simulink model "my_macro_2_2025"  (R2026a)
settings: Solver=VariableStepAuto
values from neighbouring files (symbols this model uses):
  A = [A_init, zeros(5,1) ... (first row only)    [IP_MACRO.m]    (also in testes_30_03.m)
  A_c = [A - B*K - L*C,  -B*K_i ... (first row only)    [Home1.m]
  B = [B_init ... (first row only)    [IP_MACRO.m]    (also in testes_30_03.m)
  B_c = [L ... (first row only)    [Home1.m]
  C = [C_init, zeros(2,1)]    [IP_MACRO.m]    (also in testes_30_03.m)
  C_c = -K_aug    [Home1.m]
  D = zeros(2,1)    [IP_MACRO.m]    (also in testes_30_03.m)
  D_c = [0, 0]    [Home1.m]
  x0 = [0.1 0 0.05 0 0]'    [Home1.m]
settings Model: Creator=sofia  LastModifiedBy=sofiaduarte
settings DataIOCC: SaveFormat=StructureWithTime

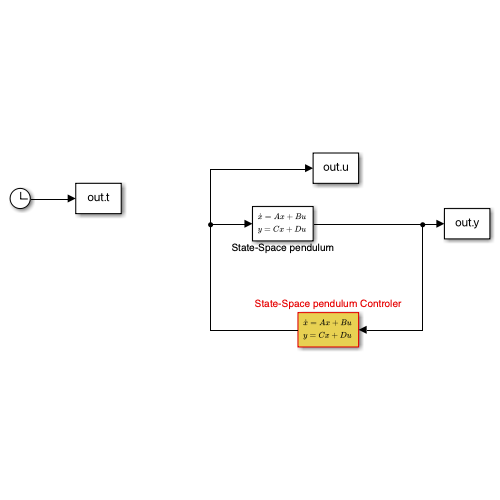
[thumbnail: Simulink's stored preview of the top-level diagram]
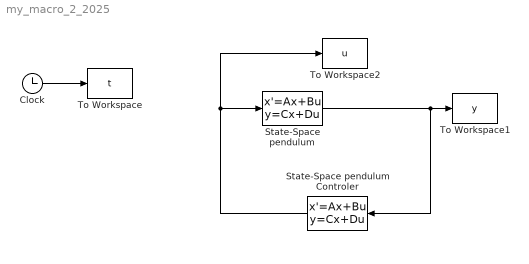
== system my_macro_2_2025 ==
  Clock : Clock
  State-Space pendulum : StateSpace  A=A  B=B  C=C  D=D  InitialCondition=x0  ContinuousStateAttributes={'x1','x2','x3','x4','x5'}
  State-Space pendulum Controler : StateSpace  A=A_c  B=B_c  C=C_c  D=D_c  InitialCondition=1
  To Workspace : ToWorkspace  VariableName=t  SampleTime=-1
  To Workspace1 : ToWorkspace  VariableName=y  SampleTime=-1
  To Workspace2 : ToWorkspace  VariableName=u  SampleTime=-1
  wires:
  State-Space pendulum/1 -> State-Space pendulum Controler/1, To Workspace1/1
  Clock/1 -> To Workspace/1
  State-Space pendulum Controler/1 -> To Workspace2/1, State-Space pendulum/1
